simulink model "sensorFusionWithControlIN1IN2"  (R2024a)
settings: Solver=FixedStepAuto  StartTime=0.0  StopTime=inf  FixedStep=motorFBRate  RelTol=1e-3
InitFcn:
  | modelParamsDD = Simulink.data.dictionary.open('modelConfigData.sldd');
  | sectModel = getSection(modelParamsDD,'Design Data');
  | contorlRate = getValue(getEntry(sectModel,'controlRate'));
  | 
  | % Complementary filter
  | fc = 10; %Hz
  | tau = 1/(2*pi*fc);
  | alpha = tau/(tau+contorlRate);
  | 
  | % Control params
  | tiltSetPoint = 1; % degree
  | D_min = 22;
  | 
  | % Tilt angle PID
  | Tw = 1;
  | b = 0.05; % lookup table
  | Kp = 35;
  | Ki = 0.005; % At 400 Hz
  | 
  | % Motor params
  | PPR = 13;
  | gearReductionRatio = 42;
  | ABPhase = 2;
  | 
  | % Motor FB params
  | motorFBRate = 0.0002; % 5 kHz
  | wToVolt = 12/(125*2*pi/60); % 125 RPM rated speed
  | Kp_m = 0.01;
  | Ki_m = 0.8;
  | Tw_m = 1;
undefined symbols (not defined in the file or in its folder): accelToUnit, angleEstRate, controlRate, gyroToUnit, MaxMotorVoltage
libraries: stm32f7xxblockslib x2
settings Model: DataDictionary=globalData.sldd  VariantConfigurationObject=RobotVariantConfig  STM32="{\"PWMOutput\":[{\"ID\":\"sensorFusionWithControlIN1IN2:205\"},{\"ID\":\"sensorFusionWithControlIN1IN2:189\"}],\"I2CControllerRead\":[{\"ID\":\"sensorFusionWithControlIN1IN2:63:801\"},{\"ID\":\"sensorFusionWithControlIN1IN2:63:802\"},{\"ID\":\"sensorFusionWithControlIN1IN2:63:803\"},{\"ID\":\"sensorFusionWithControlIN1IN2:63:804\"},{\"ID\":\"sensorFusionWithControlIN1IN2:63:799\"},{\"ID\":\"sensorFusionWithControlIN1IN2:63:800\"},{\"ID\":\"sensorFusionWithControlIN1IN2:63:813\"},{\"ID\":\"sensorFusionWithControlIN1IN2:63:814\"},{\"ID\":\"sensorFusionWithControlIN1IN2:78:799\"},{\"ID\":\"sensorFusionWithControlIN1IN2:78:800\"},{\"ID\":\"sensorFusionWithControlIN1IN2:78:801\"},{\"ID\":\"sensorFusionWithControlIN1IN2:78:802\"},{\"ID\":\"sensorFusionWithControlIN1IN2:78:803\"},{\"ID\":\"sensorFusionWithControlIN1IN2:78:804\"},{\"ID\":\"sensorFusionWithControlIN1IN2:78:812\"},{\"ID\":\"sensorFusionWithControlIN1IN2:78:813\"},{\"ID\":\"sensorFusionWithControlIN1IN2:78:814\"}],\"I2CControllerWrite\":[{\"ID\":\"sensorFusionWithControlIN1IN2:63:815\"},{\"ID\":\"sensorFusionWithControlIN1IN2:63:816\"},{\"ID\":\"sensorFusionWithControlIN1IN2:78:815\"},{\"ID\":\"sensorFusionWithControlIN1IN2:78:816\"},{\"ID\":\"sensorFusionWithControlIN1IN2:78:817\"}]}"  SimulationMode=external  Creator=Peter  LastModifiedBy=Peter
settings OptimizationCC: OptimizeBlockIOStorage=off  BufferReuse=off  ReuseModelBlockBuffer=off  GlobalBufferReuse=off  ExpressionFolding=off  EnableMemcpy=off  PassReuseOutputArgsAs=Individual arguments  LocalBlockOutputs=off  ZeroExternalMemoryAtStartup=off  ZeroInternalMemoryAtStartup=off  MaxStackSize=64  OptimizeDataStoreBuffers=off  BusAssignmentInplaceUpdate=off  OptimizationLevel=level0  OptimizationCustomize=off  EfficientTunableParamExpr=on
settings DebuggingCC: ParameterTunabilityLossMsg=error
settings HardwareCC: ProdBitPerPointer=32  ProdBitPerSizeT=32  ProdBitPerPtrDiffT=32  ProdLargestAtomicInteger=Long  ProdLargestAtomicFloat=Double  ProdWordSize=32  ProdLongLongMode=on  ProdHWDeviceType=ARM Compatible->ARM Cortex-M
settings SFSimCC: MATLABDynamicMemAlloc=off
settings RTWCC: Description=Embedded Coder  SystemTargetFile=ert.tlc  HardwareBoard=STM32F7xx Based (Single precision FPU)  TemplateMakefile=ert_default_tmf  Toolchain=GNU Tools for ARM Embedded Processors
settings CodeAppCC: GenerateComments=off  IgnoreCustomStorageClasses=off  OperatorAnnotations=on  SimulinkDataObjDesc=on  SFDataObjDesc=on  SimulinkBlockComments=off
settings ERTTargetCC: TargetLangStandard=C99 (ISO)  CodeReplacementLibrary=ARM Cortex-M  SupportComplex=off  ExtMode=on  ExtModeTransport=3  ExtModeStaticAlloc=on  ExtModeStaticAllocSize=2048  ExtModeMexFile=ext_xcp  ExtModeMexArgs=1 'COM11' 115200  ExtModeIntrfLevel=Level2 - Open

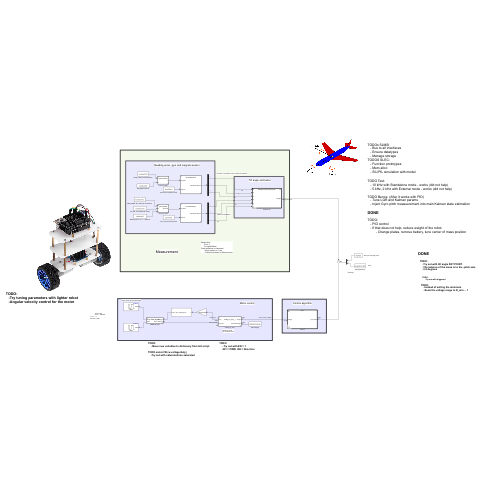
[thumbnail: Simulink's stored preview of the top-level diagram]
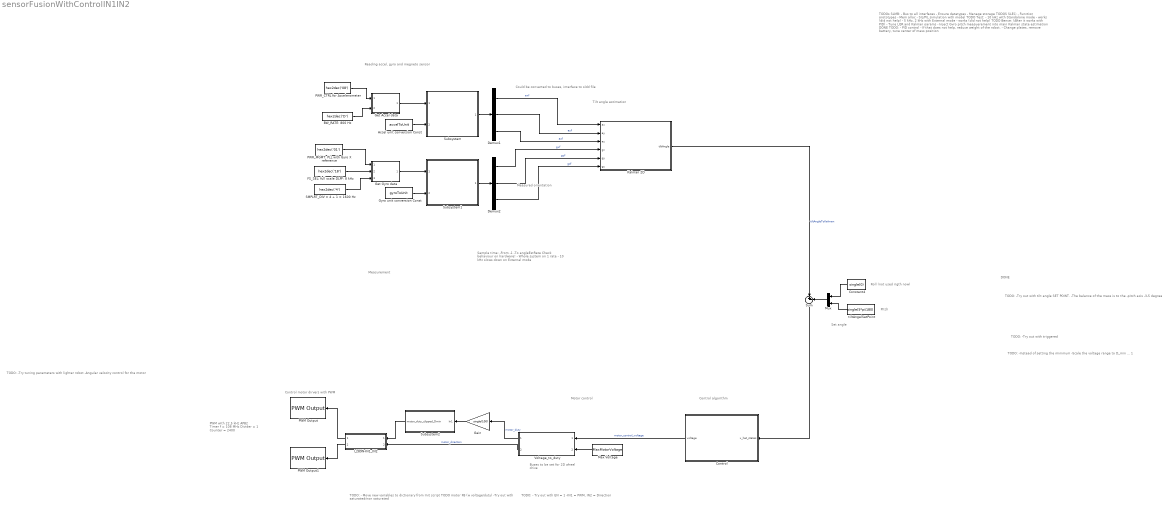
== system sensorFusionWithControlIN1IN2 ==
  note: TODO:
      | - Move new variables to dictionary from Init script
      |
      | TODO motor FB (w voltage/duty)
      | -Try out with saturated/non saturated
  note: TODO:
      | -Try tuning parameters with lighter robot
      | -Angular velocity control for the motor
  note: DONE
  note: TODO:
      | -Try out with triggered
  note: Pitch
  note: Roll (not used rigth now)
  note: Set angle
  note: TODO:
      | -Try out with tilt angle SET POINT.
      | -The balance of the mass is to the -pitch axis
      | -3-5 degrees
  note: Measured orientation
  note: TODOs SLMB:
      | - Bus to all interfaces
      | - Ensure datatypes
      | - Manage storage
      | TODOS SLEC:
      | - Function prototypes
      | - Mem alloc
      | - SIL/PIL simulation with model
      |
      | TODO Test:
      | - 10 kHz with Standalone mode - works (did not help)
      | - 5 kHz, 2 kHz with External mode - works (did not help)
      |
      | TODO Bence: (After it works with PID)
      | - Tune LQR and Kalman params
      | - Inject Gyro pitch measuerement into main Kalman state estimation
      |
      | DONE
      |
      | TODO:
      | - PID control
      | - If that does not help, reduce weight of the robot.
      | - Change plates, remove battery, tune center of mass position
  note: PWM with 22,5 kHz
      | APB2 Timer f = 108 MHz
      | Divider = 1
      | Counter = 2400
  note: Sample time:
      | -From -1
      | -To angleEstRate
      | Check behaviour on hardware!
      | - Whole system on 1 rate
      | - 10 kHz slows down on External mode
  note: Measurement
  note: Motor control
  note: Tilt angle estimation
  note: Buses to be set
      | for 2D wheel drive
  note: Control motor dirvers with PWM
  note: Could be converted to buses, interface to sldd file
  note: Reading accel, gyro and megneto sensor
  note: Control algorithm
  note: TODO:
      | -Instead of setting the minimum
      | -Scale the voltage range to D_min ... 1
  note: TODO:
      | - Try out with EN = 1
      | -IN1 = PWM, IN2 = Direction
  Accel unit conversion Const : Constant  Value=accelToUnit  OutDataTypeStr=single
  BW_RATE: 800 Hz : Constant  Value=hex2dec('D')  OutDataTypeStr=uint8
  Constant4 : Constant  Value=single(0)
  Control : Subsystem  Variant=on  VariantChoicesEnumeration=controlEnum  VariantControlVariable=controlAlgCtrl  VariantControl=Subsystem2  VariantActivationTime=inherit from Simulink.VariantControl
  Demux1 : Demux  Outputs=3
  Demux2 : Demux  Outputs=3
  FS_SEL: full scale DLPF: 8 kHz : Constant  Value=hex2dec('18')  OutDataTypeStr=uint8
  Gain : Gain  Gain=single(100)
  Get Accel data : Subsystem  TreatAsAtomicUnit=on  SystemSampleTime=angleEstRate  ReferencedSubsystem=getAccelData
  Get Gyro data : Subsystem  TreatAsAtomicUnit=on  SystemSampleTime=angleEstRate  ReferencedSubsystem=getGyroData
  Gyro unit conversion Const : Constant  Value=gyroToUnit  OutDataTypeStr=single
  Kalman 2D : Subsystem  Variant=on  VariantChoicesEnumeration=tiltEnum  VariantControlVariable=tiltEstCtrl  VariantControl=Kalman 2D  VariantActivationTime=inherit from Simulink.VariantControl
  L289N-IN1_IN2 : Subsystem  TreatAsAtomicUnit=on  SystemSampleTime=controlRate  ReferencedSubsystem=L289N_IN1_IN2
  Max Voltage : Constant  Value=MaxMotorVoltage  OutDataTypeStr=single
  Mux : Mux  Inputs=2
  PWM Output : stm32f7xxblockslib/PWM Output  TimerModule=TIM8  DutycycleUnits=Percentage  EnableChannel1=off  EnableChannel2=off  EnableChannel3=on  EnableChannel4=off  EnableChannel5=off  EnableChannel6=off  EnableCounterInput=off  EnableMainOutputInput=off  EnableFrequencyInput=off  SetRCAfterCE=off  OutputDirection=off  OutputMainOutputEnableStatus=off  SampleTime=0.1  EnableSimPort=off  EnableUpdateEvent=off  EnableCaptureCompare1Event=off  EnableCaptureCompare2Event=off  EnableCaptureCompare3Event=off  EnableCaptureCompare4Event=off  EnableTriggerEvent=off  EnableBreakEvent=off  EnableBreakEvent2=off  ProcessorFamily=STM32F7  hoistedMaskSrc=ECSoC/ECSimCodegen/PWM Output
  PWM Output1 : stm32f7xxblockslib/PWM Output  TimerModule=TIM8  DutycycleUnits=Percentage  EnableChannel1=off  EnableChannel2=off  EnableChannel3=off  EnableChannel4=on  EnableChannel5=off  EnableChannel6=off  EnableCounterInput=off  EnableMainOutputInput=off  EnableFrequencyInput=off  SetRCAfterCE=off  OutputDirection=off  OutputMainOutputEnableStatus=off  SampleTime=0.1  EnableSimPort=off  EnableUpdateEvent=off  EnableCaptureCompare1Event=off  EnableCaptureCompare2Event=off  EnableCaptureCompare3Event=off  EnableCaptureCompare4Event=off  EnableTriggerEvent=off  EnableBreakEvent=off  EnableBreakEvent2=off  ProcessorFamily=STM32F7  hoistedMaskSrc=ECSoC/ECSimCodegen/PWM Output
  PWR_CTRL for Accelerometer : Constant  Value=hex2dec('08')  OutDataTypeStr=uint8
  PWR_MGMT: PLL with Gyro X reference : Constant  Value=hex2dec('01')  OutDataTypeStr=uint8
  SMPLRT_DIV = 4 + 1 = 1600 Hz : Constant  Value=hex2dec('4')  OutDataTypeStr=uint8
  Subsystem : Subsystem  TreatAsAtomicUnit=on  SystemSampleTime=angleEstRate  ReferencedSubsystem=convertRawAccel
  Subsystem1 : Subsystem  TreatAsAtomicUnit=on  SystemSampleTime=angleEstRate  ReferencedSubsystem=convertRawGyro
  Subsystem2 : Subsystem
  Sum : Sum  Inputs=|+-
  Voltage_to_duty : Subsystem  TreatAsAtomicUnit=on  SystemSampleTime=controlRate  ReferencedSubsystem=Voltage_to_duty_1
  tiltAngelSetPoint : Constant  Value=single(5*pi/180)
  wires:
  Max Voltage/1 -> Voltage_to_duty/2
  Gyro unit conversion Const/1 -> Subsystem1/2
  Subsystem1/1 -> Demux2/1
  PWR_MGMT: PLL with Gyro X reference/1 -> Get Gyro data/1
  Get Gyro data/1 -> Subsystem1/1
  Kalman 2D/1(tiltAngle) -> Sum/1  "tiltAngleToKalman"
  Demux1/1 -> Kalman 2D/1(ax)  "axf"
  Demux1/2 -> Kalman 2D/2(ay)  "ayf"
  Demux1/3 -> Kalman 2D/3(az)  "azf"
  Demux2/3 -> Kalman 2D/6(gz)  "gzf"
  Get Accel data/1 -> Subsystem/1
  Accel unit conversion Const/1 -> Subsystem/2
  Subsystem/1 -> Demux1/1
  Control/1(voltage) -> Voltage_to_duty/1  "motor_control_voltage"
  Demux2/1 -> Kalman 2D/4(gx)  "gxf"
  Demux2/2 -> Kalman 2D/5(gy)  "gyf"
  BW_RATE: 800 Hz/1 -> Get Accel data/2
  PWR_CTRL for Accelerometer/1 -> Get Accel data/1
  FS_SEL: full scale DLPF: 8 kHz/1 -> Get Gyro data/2
  SMPLRT_DIV = 4 + 1 = 1600 Hz/1 -> Get Gyro data/3
  Sum/1 -> Control/1(x_hat_states)
  Mux/1 -> Sum/2
  Constant4/1 -> Mux/1
  tiltAngelSetPoint/1 -> Mux/2
  Voltage_to_duty/1 -> Gain/1  "motor_duty"
  Voltage_to_duty/2 -> L289N-IN1_IN2/2  "motor_direction"
  L289N-IN1_IN2/1 -> PWM Output/1
  L289N-IN1_IN2/2 -> PWM Output1/1
  Subsystem2/1(motor_duty_clipped_Dmin) -> L289N-IN1_IN2/1
  Gain/1 -> Subsystem2/1(In1)

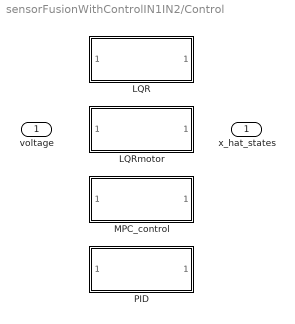
== system sensorFusionWithControlIN1IN2/Control ==
  x_hat_states : Inport  OutDataTypeStr=single
  LQR : Subsystem  TreatAsAtomicUnit=on  SystemSampleTime=controlRate  VariantControl=controlAlgCtrl == controlEnum.LQR  ReferencedSubsystem=LQR
  LQRmotor : Subsystem  TreatAsAtomicUnit=on  SystemSampleTime=controlRate  VariantControl=controlAlgCtrl == controlEnum.LQRmotor  ReferencedSubsystem=LQRmotor
  MPC_control : Subsystem  TreatAsAtomicUnit=on  SystemSampleTime=controlRate  VariantControl=controlAlgCtrl == controlEnum.MPC_control  ReferencedSubsystem=MPC_control
  PID : Subsystem  TreatAsAtomicUnit=on  SystemSampleTime=controlRate  VariantControl=controlAlgCtrl == controlEnum.PID  ReferencedSubsystem=PID
  voltage : Outport  OutDataTypeStr=single

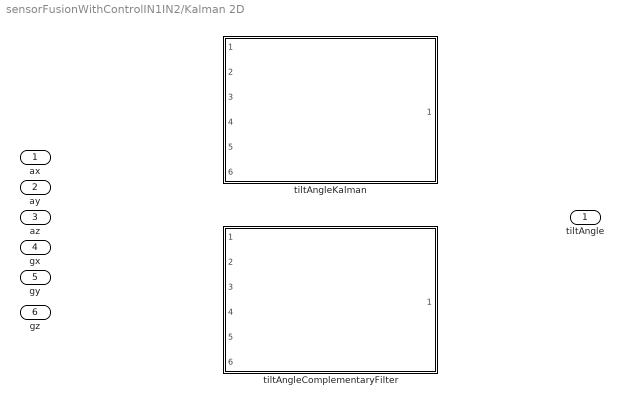
== system sensorFusionWithControlIN1IN2/Kalman 2D ==
  ax : Inport
  ay : Inport  Port=2
  az : Inport  Port=3
  gx : Inport  Port=4
  gy : Inport  Port=5
  gz : Inport  Port=6
  tiltAngleComplementaryFilter : Subsystem  TreatAsAtomicUnit=on  SystemSampleTime=controlRate  VariantControl=tiltEstCtrl == tiltEnum.tiltAngleComplementaryFilter  ReferencedSubsystem=tiltAngleComplementaryFilter
  tiltAngleKalman : Subsystem  TreatAsAtomicUnit=on  SystemSampleTime=angleEstRate  VariantControl=tiltEstCtrl == tiltEnum.tiltAngleKalman  ReferencedSubsystem=tiltAngleKalman
  tiltAngle : Outport

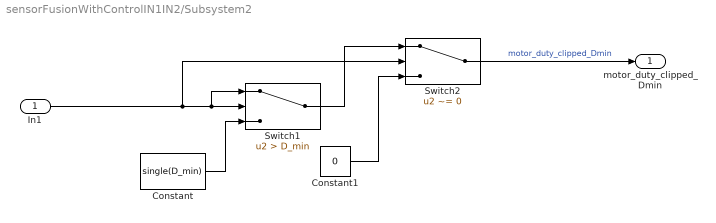
== system sensorFusionWithControlIN1IN2/Subsystem2 ==
  In1 : Inport
  Constant : Constant  Value=single(D_min)  OutDataTypeStr=single
  Constant1 : Constant  Value=0  OutDataTypeStr=single
  Switch1 : Switch  Criteria=u2 > Threshold  Threshold=D_min  OutDataTypeStr=single  SaturateOnIntegerOverflow=off  InputSameDT=off
  Switch2 : Switch  Criteria=u2 ~= 0  OutDataTypeStr=single  SaturateOnIntegerOverflow=off  InputSameDT=off
  motor_duty_clipped_Dmin : Outport
  wires:
  In1/1 -> Switch2/2, Switch1/2, Switch1/1
  Switch1/1 -> Switch2/1
  Constant1/1 -> Switch2/3
  Switch2/1 -> motor_duty_clipped_Dmin/1  "motor_duty_clipped_Dmin"
  Constant/1 -> Switch1/3
